simulink model "powertrain_model-mar"  (R2023a)
settings: Solver=VariableStepAuto  StartTime=0.0  StopTime=3500  RelTol=1e-3
values from neighbouring files (symbols this model uses):
  drivecycleData = readtable('extracted_data_filtered - Copy.csv')    [Drive_Cycle_Info.m]    (also in Old_Init.m = table2array(drivecycleData(:,2:5)); init.m = table2array(drivecycleData(:,2:5)); loadDriveCycle-mar.m = table2array(drivecycleData(:,2:5)); loadDriveCycle.m = table2array(drivecycleData(:,2:5)))
  eta_ess = 0.8    [Old_Init.m]    (also in init.m; old_script.m)
  params = table2struct(vehicleData(strcmp(vehicleData.Make, vehicleName), :))    [Old_Init.m]    (also in VehicleParamsLoader.m = loadVehicleParams(vehicleType, obj.ExcelFilePath); getVehicleParams.m = table2struct(T(strcmp(T.Make, vehicleName), :)); init.m = table2struct(T(strcmp(T.Make,'Renault Kangoo -E'), :)); loadParams.m = table2struct(T(strcmp(T.Make, targetMake), :)))
  SOC_init = 0.5    [Old_Init.m]    (also in init.m; loadVehicleParams.m; old_script.m)
undefined symbols (not defined in the file or in its folder): E_ess_max, magnitude
settings Model: Creator=cob_e  LastModifiedBy=cob_e

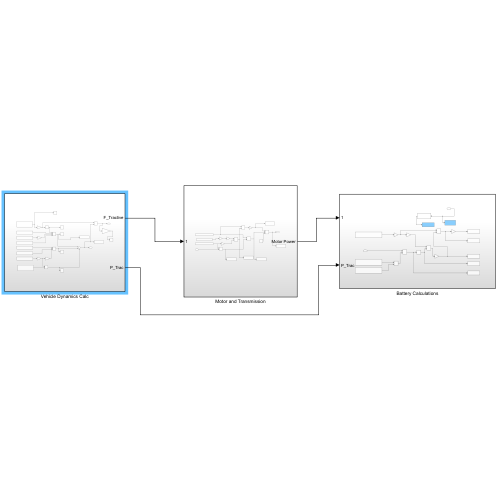
[thumbnail: Simulink's stored preview of the top-level diagram]
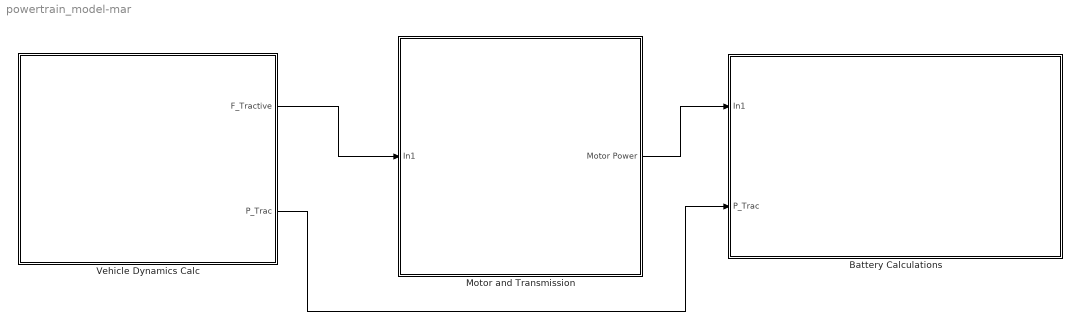
== system powertrain_model-mar ==
  Battery Calculations : Subsystem
  Motor and Transmission : Subsystem
  Vehicle Dynamics Calc : Subsystem
  wires:
  Vehicle Dynamics Calc/1(F_Tractive) -> Motor and Transmission/1(In1)
  Motor and Transmission/1(Motor Power) -> Battery Calculations/1(In1)
  Vehicle Dynamics Calc/2(P_Trac) -> Battery Calculations/2(P_Trac)

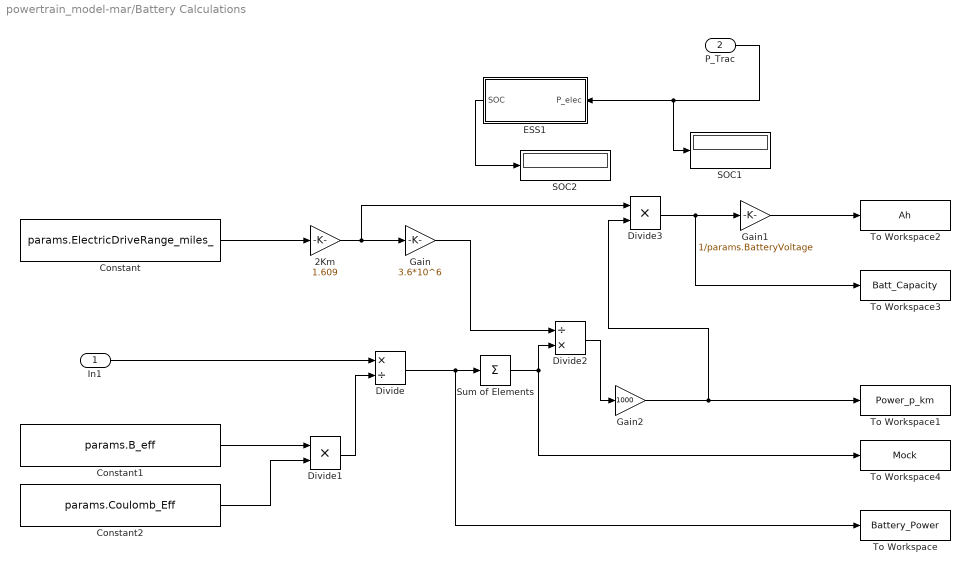
== system powertrain_model-mar/Battery Calculations ==
  In1 : Inport
  P_Trac : Inport  Port=2
  2Km : Gain  Gain=1.609
  Constant : Constant  Value=params.ElectricDriveRange_miles_
  Constant1 : Constant  Value=params.B_eff
  Constant2 : Constant  Value=params.Coulomb_Eff
  Divide : Product  Inputs=*/
  Divide1 : Product  Inputs=**
  Divide2 : Product  Inputs=/*
  Divide3 : Product  Inputs=**
  ESS1 : Subsystem  mask{E_max=E_ess_max, eta_ess=eta_ess}
      mask prompts: E_max "Maximum energy, J"; eta_ess "round-trip efficiency"
  Gain : Gain  Gain=3.6*10^6
  Gain1 : Gain  Gain=1/params.BatteryVoltage
  Gain2 : Gain  Gain=1000
  SOC1 : Display
  SOC2 : Display
  Sum of Elements : Sum  Inputs=+
  To Workspace : ToWorkspace  VariableName=Battery_Power  SaveFormat=Timeseries  SampleTime=-1
  To Workspace1 : ToWorkspace  VariableName=Power_p_km  SaveFormat=Timeseries  SampleTime=-1
  To Workspace2 : ToWorkspace  VariableName=Ah  SaveFormat=Timeseries  SampleTime=-1
  To Workspace3 : ToWorkspace  VariableName=Batt_Capacity  SaveFormat=Timeseries  SampleTime=-1
  To Workspace4 : ToWorkspace  VariableName=Mock  SaveFormat=Timeseries  SampleTime=-1
  wires:
  Sum of Elements/1 -> Divide2/2, To Workspace4/1
  Divide/1 -> Sum of Elements/1, To Workspace/1
  Gain/1 -> Divide2/1
  In1/1 -> Divide/1
  Gain1/1 -> To Workspace2/1
  Divide3/1 -> To Workspace3/1, Gain1/1
  Divide2/1 -> Gain2/1
  Gain2/1 -> To Workspace1/1, Divide3/2
  Constant1/1 -> Divide1/1
  Constant2/1 -> Divide1/2
  Divide1/1 -> Divide/2
  2Km/1 -> Divide3/1, Gain/1
  Constant/1 -> 2Km/1
  P_Trac/1 -> SOC1/1, ESS1/1(P_elec)
  ESS1/1(SOC) -> SOC2/1

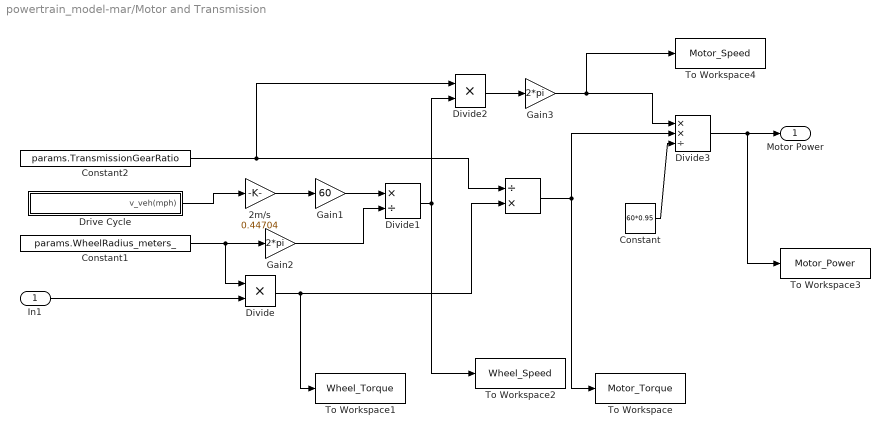
== system powertrain_model-mar/Motor and Transmission ==
  In1 : Inport
  " " : Product  Inputs=/*
  2m/s : Gain  Gain=0.44704
  Constant : Constant  Value=60*0.95
  Constant1 : Constant  Value=params.WheelRadius_meters_
  Constant2 : Constant  Value=params.TransmissionGearRatio
  Divide : Product  Inputs=**
  Divide1 : Product  Inputs=*/
  Divide2 : Product  Inputs=**  RndMeth=Zero  SaturateOnIntegerOverflow=on
  Divide3 : Product  Inputs=**/
  Drive Cycle : Subsystem  mask{schedule=drivecycleData}
      mask prompts: schedule "drive schedule"
      mask init:
      | N=length(schedule(:,1))
  Gain1 : Gain  Gain=60
  Gain2 : Gain  Gain=2*pi
  Gain3 : Gain  Gain=2*pi
  To Workspace : ToWorkspace  VariableName=Motor_Torque  SaveFormat=Timeseries  SampleTime=-1
  To Workspace1 : ToWorkspace  VariableName=Wheel_Torque  SaveFormat=Timeseries  SampleTime=-1
  To Workspace2 : ToWorkspace  VariableName=Wheel_Speed  SaveFormat=Timeseries  SampleTime=-1
  To Workspace3 : ToWorkspace  VariableName=Motor_Power  SaveFormat=Timeseries  SampleTime=-1
  To Workspace4 : ToWorkspace  VariableName=Motor_Speed  SaveFormat=Timeseries  SampleTime=-1
  Motor Power : Outport
  wires:
  Divide2/1 -> Gain3/1
  Constant/1 -> Divide3/3
  Constant2/1 -> " "/1, Divide2/1
  Divide3/1 -> To Workspace3/1, Motor Power/1
  Divide1/1 -> To Workspace2/1, Divide2/2
  Constant1/1 -> Divide/1, Gain2/1
  Gain2/1 -> Divide1/2
  Gain3/1 -> To Workspace4/1, Divide3/1
  " "/1 -> To Workspace/1, Divide3/2
  Gain1/1 -> Divide1/1
  2m/s/1 -> Gain1/1
  Drive Cycle/1(v_veh(mph)) -> 2m/s/1
  Divide/1 -> To Workspace1/1, " "/2
  In1/1 -> Divide/2

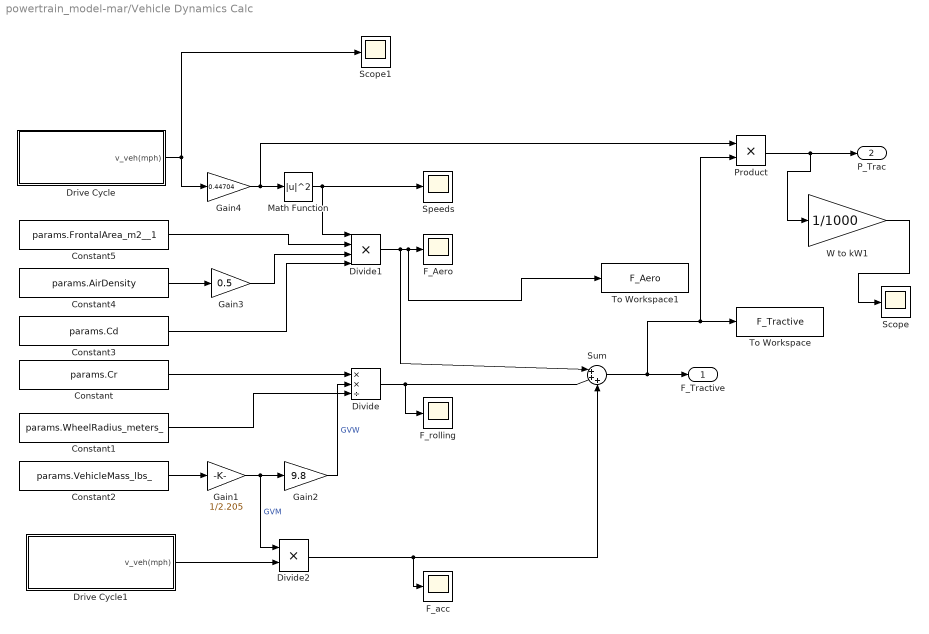
== system powertrain_model-mar/Vehicle Dynamics Calc ==
  Constant : Constant  Value=params.Cr
  Constant1 : Constant  Value=params.WheelRadius_meters_
  Constant2 : Constant  Value=params.VehicleMass_lbs_
  Constant3 : Constant  Value=params.Cd
  Constant4 : Constant  Value=params.AirDensity
  Constant5 : Constant  Value=params.FrontalArea_m2__1
  Divide : Product  Inputs=**/
  Divide1 : Product  Inputs=****
  Divide2 : Product  Inputs=**
  Drive Cycle : Subsystem  mask{schedule=drivecycleData}
      mask prompts: schedule "drive schedule"
      mask init:
      | N=length(schedule(:,1))
  Drive Cycle1 : Subsystem  mask{schedule=drivecycleData}
      mask prompts: schedule "drive schedule"
      mask init:
      | N=length(schedule(:,1))
  F_Aero : Scope
  F_acc : Scope
  F_rolling : Scope
  Gain1 : Gain  Gain=1/2.205
  Gain2 : Gain  Gain=9.8
  Gain3 : Gain  Gain=0.5
  Gain4 : Gain  Gain=0.44704
  Math Function : Math  Operator=magnitude^2
  Product : Product
  Scope : Scope
  Scope1 : Scope
  Speeds : Scope
  Sum : Sum  Inputs=|+++
  To Workspace : ToWorkspace  VariableName=F_Tractive  SaveFormat=Timeseries  SampleTime=-1
  To Workspace1 : ToWorkspace  VariableName=F_Aero  SaveFormat=Timeseries  SampleTime=-1
  W to kW1 : Gain  Gain=1/1000
  F_Tractive : Outport
  P_Trac : Outport  Port=2
  wires:
  Divide/1 -> Sum/2, F_rolling/1
  Constant2/1 -> Gain1/1
  Constant4/1 -> Gain3/1
  Constant/1 -> Divide/1
  Divide1/1 -> Sum/1, To Workspace1/1, F_Aero/1
  Gain3/1 -> Divide1/3
  Gain2/1 -> Divide/2  "GVW"
  Gain1/1 -> Divide2/1, Gain2/1  "GVM"
  Drive Cycle/1(v_veh(mph)) -> Scope1/1, Gain4/1
  Constant5/1 -> Divide1/2
  Constant3/1 -> Divide1/4
  Divide2/1 -> Sum/3, F_acc/1
  Sum/1 -> Product/2, To Workspace/1, F_Tractive/1
  Gain4/1 -> Product/1, Math Function/1
  Math Function/1 -> Divide1/1, Speeds/1
  Constant1/1 -> Divide/3
  Product/1 -> W to kW1/1, P_Trac/1
  W to kW1/1 -> Scope/1
  Drive Cycle1/1(v_veh(mph)) -> Divide2/2

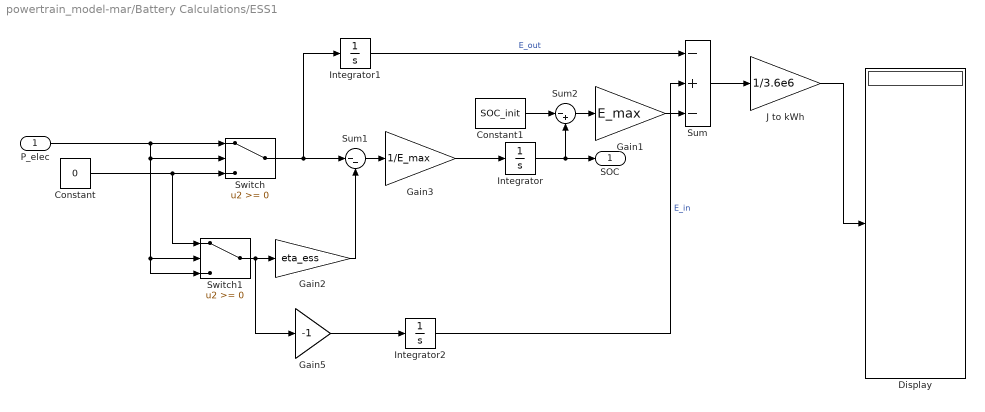
== system powertrain_model-mar/Battery Calculations/ESS1 ==
  P_elec : Inport
  Constant : Constant  Value=0
  Constant1 : Constant  Value=SOC_init
  Display : Display
  Gain1 : Gain  Gain=E_max  OutDataTypeStr=fixdt('double', 'DataTypeOverride', 'Off')
  Gain2 : Gain  Gain=eta_ess
  Gain3 : Gain  Gain=1/E_max  OutDataTypeStr=fixdt('double', 'DataTypeOverride', 'Off')
  Gain5 : Gain  Gain=-1  OutDataTypeStr=fixdt('double', 'DataTypeOverride', 'Off')
  Integrator : Integrator  InitialCondition=SOC_init  LimitOutput=on  UpperSaturationLimit=1  LowerSaturationLimit=0
  Integrator1 : Integrator
  Integrator2 : Integrator
  J to kWh : Gain  Gain=1/3.6e6  OutDataTypeStr=fixdt('double', 'DataTypeOverride', 'Off')
  Sum : Sum  Inputs=-+-
  Sum1 : Sum  Inputs=|--
  Sum2 : Sum  Inputs=|-+
  Switch : Switch  OutDataTypeStr=double  SaturateOnIntegerOverflow=off  InputSameDT=off
  Switch1 : Switch  OutDataTypeStr=double  SaturateOnIntegerOverflow=off  InputSameDT=off
  SOC : Outport
  wires:
  P_elec/1 -> Switch1/2, Switch1/3, Switch/2, Switch/1
  Gain3/1 -> Integrator/1
  Gain2/1 -> Sum1/2
  Switch1/1 -> Gain5/1, Gain2/1
  Sum1/1 -> Gain3/1
  Constant/1 -> Switch1/1, Switch/3
  Integrator/1 -> Sum2/2, SOC/1
  Switch/1 -> Integrator1/1, Sum1/1
  Integrator1/1 -> Sum/1  "E_out"
  Integrator2/1 -> Sum/2  "E_in"
  Constant1/1 -> Sum2/1
  Sum2/1 -> Gain1/1
  Gain1/1 -> Sum/3
  Sum/1 -> J to kWh/1
  J to kWh/1 -> Display/1
  Gain5/1 -> Integrator2/1

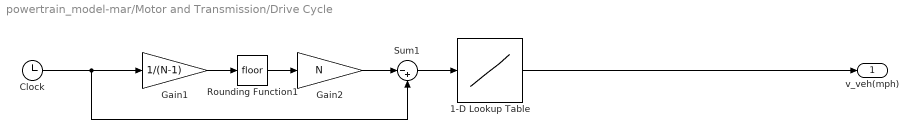
== system powertrain_model-mar/Motor and Transmission/Drive Cycle ==
  1-D Lookup Table : Lookup_n-D  NumberOfTableDimensions=1  BreakpointsForDimension1=schedule(:,1)  Table=schedule(:,3)  InternalRulePriority=Speed  RndMeth=Simplest
  Clock : Clock
  Gain1 : Gain  Gain=1/(N-1)
  Gain2 : Gain  Gain=N
  Rounding Function1 : Rounding
  Sum1 : Sum  Inputs=|-+
  v_veh(mph) : Outport  VectorParamsAs1DForOutWhenUnconnected=off
  wires:
  Clock/1 -> Gain1/1, Sum1/2
  Sum1/1 -> 1-D Lookup Table/1
  Gain2/1 -> Sum1/1
  Rounding Function1/1 -> Gain2/1
  Gain1/1 -> Rounding Function1/1
  1-D Lookup Table/1 -> v_veh(mph)/1

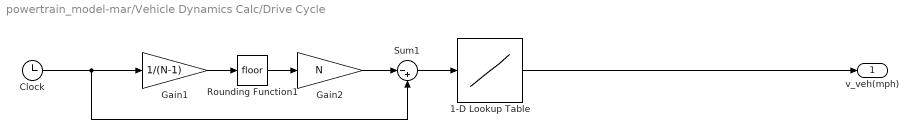
== system powertrain_model-mar/Vehicle Dynamics Calc/Drive Cycle ==
  1-D Lookup Table : Lookup_n-D  NumberOfTableDimensions=1  BreakpointsForDimension1=schedule(:,1)  Table=schedule(:,3)  InternalRulePriority=Speed  RndMeth=Simplest
  Clock : Clock
  Gain1 : Gain  Gain=1/(N-1)
  Gain2 : Gain  Gain=N
  Rounding Function1 : Rounding
  Sum1 : Sum  Inputs=|-+
  v_veh(mph) : Outport  VectorParamsAs1DForOutWhenUnconnected=off
  wires:
  Clock/1 -> Gain1/1, Sum1/2
  Sum1/1 -> 1-D Lookup Table/1
  Gain2/1 -> Sum1/1
  Rounding Function1/1 -> Gain2/1
  Gain1/1 -> Rounding Function1/1
  1-D Lookup Table/1 -> v_veh(mph)/1

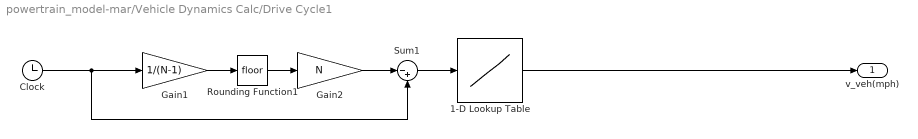
== system powertrain_model-mar/Vehicle Dynamics Calc/Drive Cycle1 ==
  1-D Lookup Table : Lookup_n-D  NumberOfTableDimensions=1  BreakpointsForDimension1=schedule(:,1)  Table=schedule(:,4)  InternalRulePriority=Speed  RndMeth=Simplest
  Clock : Clock
  Gain1 : Gain  Gain=1/(N-1)
  Gain2 : Gain  Gain=N
  Rounding Function1 : Rounding
  Sum1 : Sum  Inputs=|-+
  v_veh(mph) : Outport  VectorParamsAs1DForOutWhenUnconnected=off
  wires:
  Clock/1 -> Gain1/1, Sum1/2
  Sum1/1 -> 1-D Lookup Table/1
  Gain2/1 -> Sum1/1
  Rounding Function1/1 -> Gain2/1
  Gain1/1 -> Rounding Function1/1
  1-D Lookup Table/1 -> v_veh(mph)/1
